simulink model "problem2"  (R2020b)
settings: Solver=VariableStepAuto  StartTime=0.0  StopTime=100.0  RelTol=1e-3
undefined symbols (not defined in the file): b, K1, K2, M1, M2
settings Model: Creator=admin  LastModifiedBy=admin
settings DataIOCC: ExternalInput=[t, inputsignal]  LoadExternalInput=on

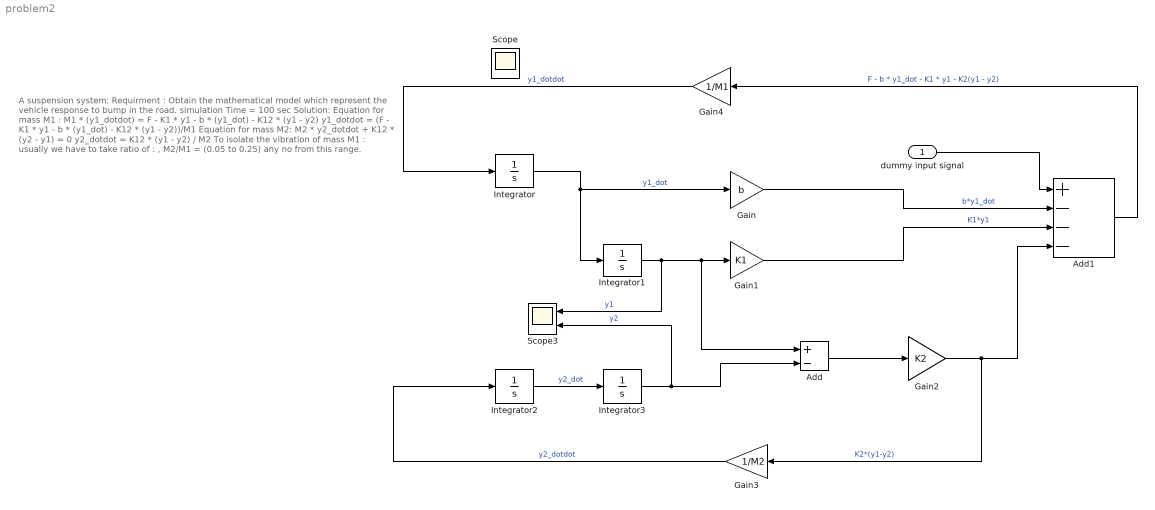
== system problem2 ==
  note: A suspension system:
      |
      | Requirment :
      | Obtain the mathematical model which represent the vehicle response to bump in the road.
      | simulation Time = 100 sec
      |
      | Solution:
      | Equation for mass M1 :
      | M1 * (y1_dotdot) = F - K1 * y1 - b * (y1_dot) - K12 * (y1 - y2)
      |
      | y1_dotdot = (F - K1 * y1 - b * (y1_dot) - K12 * (y1 - y2))/M1
      |
      | Equation for mass M2:
      | M2 * y2_dotdot + K12 * (y2 - y1) = 0
      |
      | y2_dotdot = K12 * (y1 - y2) / M2
      |
      | To isolate the vibration of mass M1 :
      | usually we have to take ratio of : , M2/M1 = (0.05 to 0.25) any no from this range.
  "dummy input signal " : Inport
  Add : Sum  Inputs=+-
  Add1 : Sum  Inputs=+---
  Gain : Gain  Gain=b
  Gain1 : Gain  Gain=K1
  Gain2 : Gain  Gain=K2
  Gain3 : Gain  Gain=1/M2
  Gain4 : Gain  Gain=1/M1
  Integrator{,1..3} (4 alike) : Integrator
  Scope3 : Scope  NumInputPorts=2
  Scope : Scope
  wires:
  Integrator/1 -> Integrator1/1, Gain/1  "y1_dot"
  Gain4/1 -> Integrator/1  "y1_dotdot"
  Integrator1/1 -> Scope3/1, Gain1/1, Add/1  "y1"
  Integrator2/1 -> Integrator3/1  "y2_dot"
  Integrator3/1 -> Scope3/2, Add/2  "y2"
  Gain/1 -> Add1/2  "b*y1_dot"
  Gain1/1 -> Add1/3  "K1*y1"
  Add/1 -> Gain2/1
  Gain2/1 -> Add1/4, Gain3/1  "K2*(y1-y2)"
  Gain3/1 -> Integrator2/1  "y2_dotdot"
  Add1/1 -> Gain4/1  "F - b * y1_dot - K1 * y1 - K2(y1 - y2)"
  "dummy input signal "/1 -> Add1/1
